simulink model "Model5DOF"  (R2020a)
settings: Solver=FixedStepAuto  StartTime=0.0  StopTime=200  FixedStep=0.01  RelTol=1e-3
libraries: simulink x5, vrlib x3
settings Model: Creator=DaseonHong  LastModifiedBy=fdcl

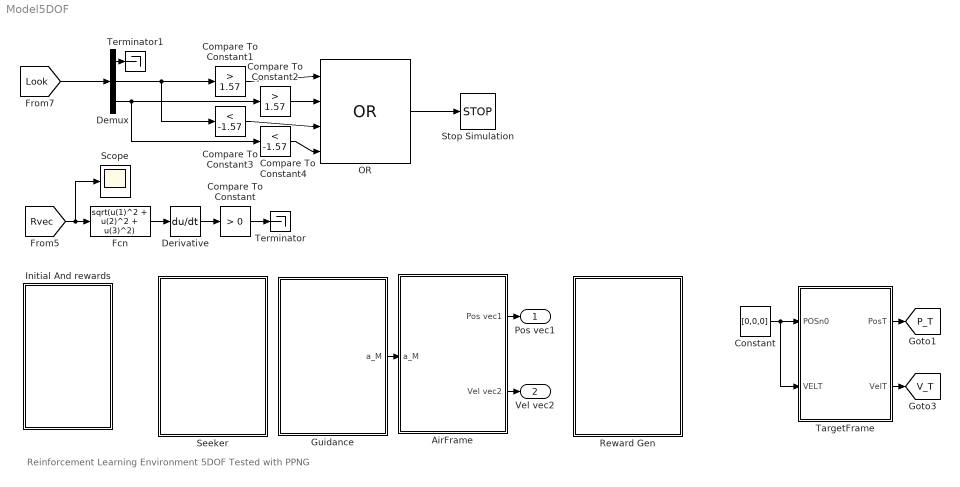
== system Model5DOF ==
  note: Reinforcement Learning Environment
      | 5DOF
      | Tested with PPNG
  AirFrame : Subsystem
  Compare To Constant : simulink/Logic and Bit Operations/Compare To Constant  relop=>  const=0  OutDataTypeStr=boolean
  Compare To Constant1 : simulink/Logic and Bit Operations/Compare To Constant  relop=>  const=1.57  OutDataTypeStr=boolean
  Compare To Constant2 : simulink/Logic and Bit Operations/Compare To Constant  relop=>  const=1.57  OutDataTypeStr=boolean
  Compare To Constant3 : simulink/Logic and Bit Operations/Compare To Constant  relop=<  const=-1.57  OutDataTypeStr=boolean
  Compare To Constant4 : simulink/Logic and Bit Operations/Compare To Constant  relop=<  const=-1.57  OutDataTypeStr=boolean
  Constant : Constant  Value=[0,0,0]
  Demux : Demux  Outputs=3
  Derivative : Derivative
  Fcn : Fcn  Expr=sqrt(u(1)^2 + u(2)^2 + u(3)^2)
  Guidance : Subsystem
  Initial And rewards : Subsystem  mask{Parameter1=90, Parameter2=10, Parameter5=10000, Parameter6=10000, Parameter7=0, Parameter8=0, Parameter4=280, Parameter15=3, Parameter9=-10000, Parameter10=5000, Parameter19=-1000, Parameter21=0, Parameter11=280, Parameter16=3, Parameter12=0, Parameter13=0, Parameter20=-1000, Parameter23=0}
      mask prompts: Parameter1 "Impact time"; Parameter2 "delayed fire"; Parameter5 "targetposx"; Parameter6 "targetposy"; Parameter7 "targetvelx"; Parameter8 "targetvely"; Parameter4 "speed"; Parameter15 "PNGcoeff"; Parameter9 "initposx"; Parameter10 "initposy"; Parameter19 "initposz"; Parameter21 "initpsi"; Parameter11 "speed"; Parameter16 "PNGcoeff"; Parameter12 "initposx"; Parameter13 "initposy"; Parameter20 "initposz"; Parameter23 "initpsi"
      mask init:
      | td      = Parameter1;
      | LaunchD = Parameter2;
      | x_t     = Parameter5;
      | y_t     = Parameter6;
      | vx_t    = Parameter7;
      | vy_t    = Parameter8;
      | 
      | SoM     = Parameter4;
      | Nval    = Parameter15;
      | x_m1    = Parameter9;
      | y_m1    = Parameter10;
      | z_m1    = Parameter19;
      | psi0    = Parameter21;
      | 
      | SoM2    = Parameter11;
      | Nval2   = Parameter16;
      | x_m2    = Parameter12;
      | y_m2    = Parameter13;
      | z_m2    = Parameter20;
      | psi20   = Parameter23;
      mask TypeOptions Parameter15: 1 | 2 | 3 | 4 | 5
      mask TypeOptions Parameter16: 1 | 2 | 3 | 4 | 5
      mask DialogControl Container4 Prompt: Common Param
      mask DialogControl Container7 Prompt: Time
      mask DialogControl Container11 Prompt: Target
      mask DialogControl Container5 Prompt: Missile 1
      mask DialogControl Container8 Prompt: Missile 2
  OR : Logic  Operator=OR  Inputs=4  IconShape=distinctive  AllPortsSameDT=off  OutDataTypeStr=boolean
  Reward Gen : Subsystem
  Scope : Scope
  Seeker : Subsystem
  Stop Simulation : Stop
  TargetFrame : Subsystem
      mask Display: image('$imagefile'); % Use "Edit Image" on toolstrip to change.
  Terminator : Terminator
  Terminator1 : Terminator
  Pos vec1 : Outport  VectorParamsAs1DForOutWhenUnconnected=off
  Vel vec2 : Outport  Port=2  VectorParamsAs1DForOutWhenUnconnected=off
  tag scope: P_T=global, V_T=global
  wires:
  Guidance/1(a_M) -> AirFrame/1(a_M)
  AirFrame/1(Pos vec1) -> Pos vec1/1
  AirFrame/2(Vel vec2) -> Vel vec2/1
  TargetFrame/2(VelT) -> [V_T]
  Constant/1 -> TargetFrame/2(VELT), TargetFrame/1(POSn0)
  TargetFrame/1(PosT) -> [P_T]
  [Rvec] -> Scope/1, Fcn/1
  Fcn/1 -> Derivative/1
  Compare To Constant/1 -> Terminator/1
  Derivative/1 -> Compare To Constant/1
  [Look] -> Demux/1
  Demux/1 -> Terminator1/1
  Demux/2 -> Compare To Constant3/1, Compare To Constant1/1
  Compare To Constant1/1 -> OR/1
  Compare To Constant2/1 -> OR/2
  Demux/3 -> Compare To Constant2/1, Compare To Constant4/1
  OR/1 -> Stop Simulation/1
  Compare To Constant3/1 -> OR/3
  Compare To Constant4/1 -> OR/4

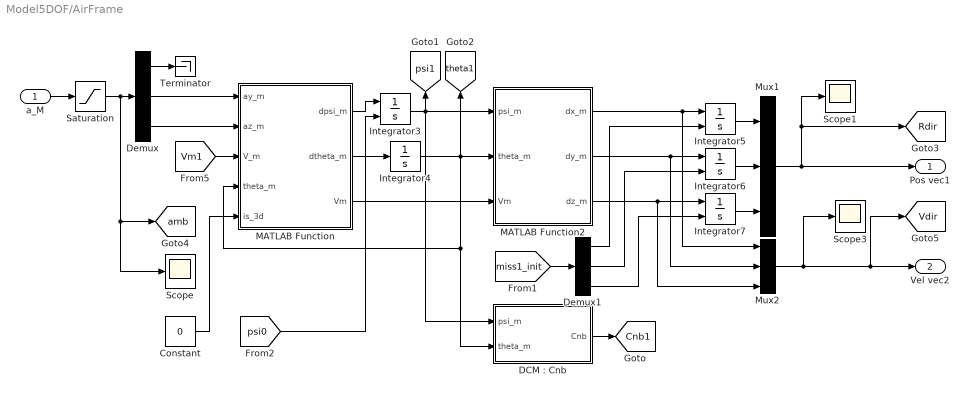
== system Model5DOF/AirFrame ==
  a_M : Inport
  Constant : Constant  Value=0
  "DCM : Cnb" : MATLAB Function  TreatAsAtomicUnit=on
  Demux : Demux  Outputs=3
  Demux1 : Demux  Outputs=3
  Integrator{3,5..7} (4 alike) : Integrator  InitialConditionSource=external
  Integrator4 : Integrator
  MATLAB Function : MATLAB Function  TreatAsAtomicUnit=on
  MATLAB Function2 : MATLAB Function  TreatAsAtomicUnit=on
  Mux1 : Mux  Inputs=3
  Mux2 : Mux  Inputs=3
  Saturation : Saturate  UpperLimit=[0;99;99]  LowerLimit=[0;-99;-99]  LinearizeAsGain=off  ZeroCross=off
  Scope : Scope
  Scope1 : Scope
  Scope3 : Scope
  Terminator : Terminator
  Pos vec1 : Outport  VectorParamsAs1DForOutWhenUnconnected=off
  Vel vec2 : Outport  Port=2  VectorParamsAs1DForOutWhenUnconnected=off
  tag scope: Cnb1=global, Rdir=global, Vdir=global, amb=global, psi1=global, theta1=global
  wires:
  MATLAB Function/1(dpsi_m) -> Integrator3/1
  Integrator7/1 -> Mux1/3
  "DCM : Cnb"/1(Cnb) -> [Cnb1]
  Constant/1 -> MATLAB Function/5(is_3d)
  [Vm1] -> MATLAB Function/3(V_m)
  Mux2/1 -> [Vdir], Vel vec2/1, Scope3/1
  Demux1/3 -> Integrator7/2
  Saturation/1 -> [amb], Scope/1, Demux/1
  Demux/3 -> MATLAB Function/2(az_m)
  MATLAB Function/3(Vm) -> MATLAB Function2/3(Vm)
  [psi0] -> Integrator3/2
  MATLAB Function/2(dtheta_m) -> Integrator4/1
  Integrator5/1 -> Mux1/1
  Demux1/2 -> Integrator6/2
  MATLAB Function2/2(dy_m) -> Mux2/2, Integrator6/1
  Demux/2 -> MATLAB Function/1(ay_m)
  Integrator3/1 -> "DCM : Cnb"/1(psi_m), MATLAB Function2/1(psi_m), [psi1]
  MATLAB Function2/3(dz_m) -> Mux2/3, Integrator7/1
  Integrator4/1 -> "DCM : Cnb"/2(theta_m), MATLAB Function/4(theta_m), MATLAB Function2/2(theta_m), [theta1]
  MATLAB Function2/1(dx_m) -> Mux2/1, Integrator5/1
  [miss1_init] -> Demux1/1
  Demux/1 -> Terminator/1
  a_M/1 -> Saturation/1
  Integrator6/1 -> Mux1/2
  Mux1/1 -> Scope1/1, [Rdir], Pos vec1/1
  Demux1/1 -> Integrator5/2

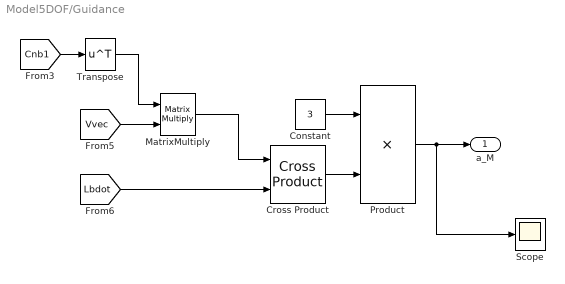
== system Model5DOF/Guidance ==
  Constant : Constant  Value=3
  Cross Product : vrlib/Utilities/Cross Product
  MatrixMultiply : Product  Multiplication=Matrix(*)
  Product : Product
  Scope : Scope
  Transpose : Math  Operator=transpose  SaturateOnIntegerOverflow=on
  a_M : Outport
  wires:
  Product/1 -> Scope/1, a_M/1
  [Vvec] -> MatrixMultiply/2
  Cross Product/1 -> Product/2
  Constant/1 -> Product/1
  [Lbdot] -> Cross Product/2
  [Cnb1] -> Transpose/1
  Transpose/1 -> MatrixMultiply/1
  MatrixMultiply/1 -> Cross Product/1

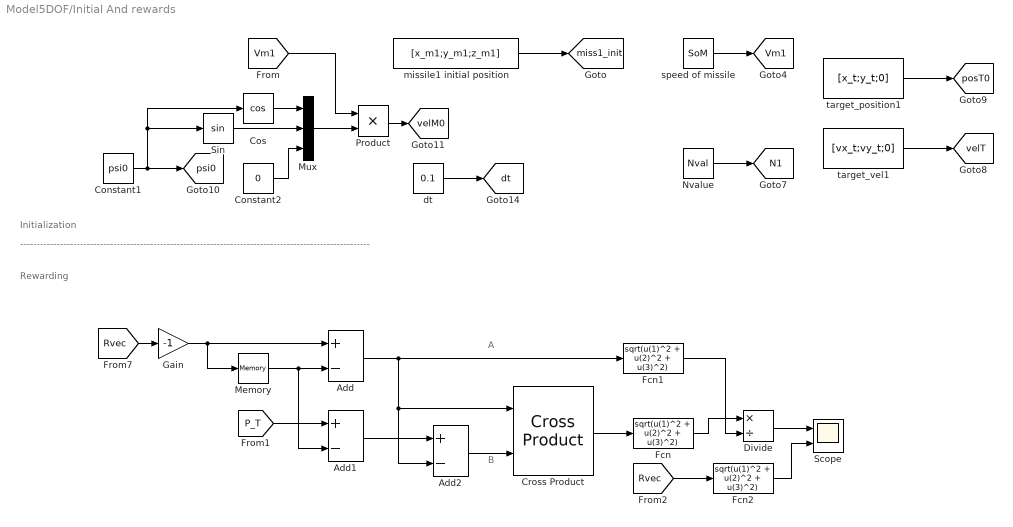
== system Model5DOF/Initial And rewards ==
  note: A
  note: Initialization
  note: ---------------------------------------------------------------------------------------------------------
  note: Rewarding
  note: B
  Add : Sum  Inputs=+-
  Add1 : Sum  Inputs=+-
  Add2 : Sum  Inputs=+-
  Constant1 : Constant  Value=psi0
  Constant2 : Constant  Value=0
  Cos : Trigonometry  Operator=cos
  Cross Product : vrlib/Utilities/Cross Product
  Divide : Product  Inputs=*/
  Fcn : Fcn  Expr=sqrt(u(1)^2 + u(2)^2 + u(3)^2)
  Fcn1 : Fcn  Expr=sqrt(u(1)^2 + u(2)^2 + u(3)^2)
  Fcn2 : Fcn  Expr=sqrt(u(1)^2 + u(2)^2 + u(3)^2)
  Gain : Gain  Gain=-1
  Memory : Memory  InitialCondition=[x_m1;y_m1;z_m1]  LinearizeAsDelay=on
  Mux : Mux  Inputs=3
  Nvalue : Constant  Value=Nval
  Product : Product
  Scope : Scope  NumInputPorts=2
  Sin : Trigonometry
  dt : Constant  Value=0.1
  missile1 initial position : Constant  Value=[x_m1;y_m1;z_m1]
  speed of missile : Constant  Value=SoM
  target_position1 : Constant  Value=[x_t;y_t;0]
  target_vel1 : Constant  Value=[vx_t;vy_t;0]
  tag scope: N1=global, Vm1=global, dt=global, miss1_init=global, posT0=global, psi0=global, velM0=global, velT=global
  wires:
  target_vel1/1 -> [velT]
  target_position1/1 -> [posT0]
  speed of missile/1 -> [Vm1]
  Nvalue/1 -> [N1]
  missile1 initial position/1 -> [miss1_init]
  Constant1/1 -> [psi0], Cos/1, Sin/1
  Mux/1 -> Product/2
  [Vm1] -> Product/1
  Sin/1 -> Mux/2
  Cos/1 -> Mux/1
  Product/1 -> [velM0]
  Constant2/1 -> Mux/3
  dt/1 -> [dt]
  [Rvec] -> Gain/1
  Gain/1 -> Add/1, Memory/1
  Memory/1 -> Add1/2, Add/2
  [P_T] -> Add1/1
  Add1/1 -> Add2/1
  Add/1 -> Cross Product/1, Add2/2, Fcn1/1
  Add2/1 -> Cross Product/2
  Cross Product/1 -> Fcn/1
  Fcn/1 -> Divide/1
  Fcn1/1 -> Divide/2
  Divide/1 -> Scope/1
  [Rvec] -> Fcn2/1
  Fcn2/1 -> Scope/2

== system Model5DOF/Reward Gen ==

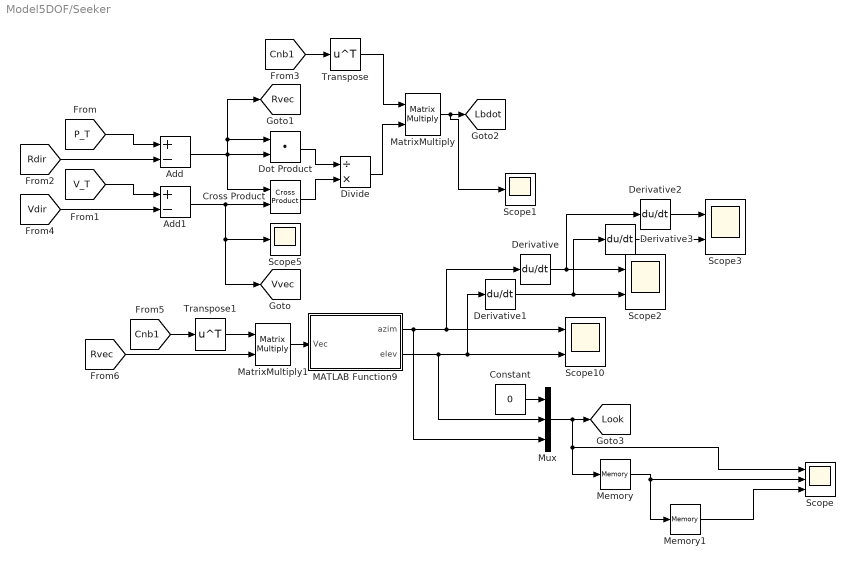
== system Model5DOF/Seeker ==
  Add : Sum  Inputs=+-
  Add1 : Sum  Inputs=+-
  Constant : Constant  Value=0
  Cross Product : vrlib/Utilities/Cross Product
  Derivative{,1..3} (4 alike) : Derivative
  Divide : Product  Inputs=/*
  Dot Product : DotProduct  InputSameDT=on  OutDataTypeStr=Inherit: Inherit via internal rule
  MATLAB Function9 : MATLAB Function  TreatAsAtomicUnit=on
  MatrixMultiply : Product  Multiplication=Matrix(*)
  MatrixMultiply1 : Product  Multiplication=Matrix(*)
  Memory : Memory  LinearizeAsDelay=on
  Memory1 : Memory  LinearizeAsDelay=on
  Mux : Mux  Inputs=3
  Scope : Scope  NumInputPorts=3
  Scope1 : Scope
  Scope10 : Scope  NumInputPorts=2
  Scope2 : Scope  NumInputPorts=2
  Scope3 : Scope  NumInputPorts=2
  Scope5 : Scope
  Transpose : Math  Operator=transpose  SaturateOnIntegerOverflow=on
  Transpose1 : Math  Operator=transpose  SaturateOnIntegerOverflow=on
  tag scope: Lbdot=global, Look=global, Rvec=global, Vvec=global
  wires:
  Dot Product/1 -> Divide/1
  Add/1 -> Cross Product/1, Dot Product/2, [Rvec], Dot Product/1
  [P_T] -> Add/1
  Add1/1 -> Cross Product/2, [Vvec], Scope5/1
  Cross Product/1 -> Divide/2
  [V_T] -> Add1/1
  [Rdir] -> Add/2
  [Vdir] -> Add1/2
  [Cnb1] -> Transpose/1
  Transpose/1 -> MatrixMultiply/1
  Divide/1 -> MatrixMultiply/2
  MatrixMultiply/1 -> Scope1/1, [Lbdot]
  MATLAB Function9/2(elev) -> Mux/2, Derivative1/1, Scope10/2
  MATLAB Function9/1(azim) -> Mux/3, Derivative/1, Scope10/1
  [Cnb1] -> Transpose1/1
  Transpose1/1 -> MatrixMultiply1/1
  MatrixMultiply1/1 -> MATLAB Function9/1(Vec)
  [Rvec] -> MatrixMultiply1/2
  Derivative/1 -> Derivative2/1, Scope2/1
  Derivative1/1 -> Derivative3/1, Scope2/2
  Derivative2/1 -> Scope3/1
  Derivative3/1 -> Scope3/2
  Constant/1 -> Mux/1
  Mux/1 -> Scope/1, Memory/1, [Look]
  Memory/1 -> Memory1/1, Scope/2
  Memory1/1 -> Scope/3

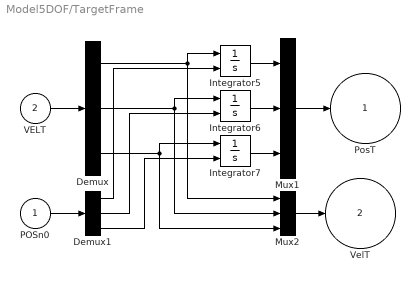
== system Model5DOF/TargetFrame ==
  POSn0 : Inport
  VELT : Inport  Port=2
  Demux : Demux  Outputs=3
  Demux1 : Demux  Outputs=3
  Integrator5 : Integrator  InitialConditionSource=external
  Integrator6 : Integrator  InitialConditionSource=external
  Integrator7 : Integrator  InitialConditionSource=external
  Mux1 : Mux  Inputs=3
  Mux2 : Mux  Inputs=3
  PosT : Outport  VectorParamsAs1DForOutWhenUnconnected=off
  VelT : Outport  Port=2  VectorParamsAs1DForOutWhenUnconnected=off
  wires:
  POSn0/1 -> Demux1/1
  Demux1/1 -> Integrator5/2
  Demux1/2 -> Integrator6/2
  Demux1/3 -> Integrator7/2
  Integrator5/1 -> Mux1/1
  Integrator6/1 -> Mux1/2
  Integrator7/1 -> Mux1/3
  Mux1/1 -> PosT/1
  Demux/2 -> Integrator6/1, Mux2/2
  Demux/3 -> Integrator7/1, Mux2/3
  Mux2/1 -> VelT/1
  Demux/1 -> Integrator5/1, Mux2/1
  VELT/1 -> Demux/1

== matlab function Model5DOF/AirFrame/DCM : Cnb ==
  data: psi_m input; Cnb output; theta_m input
function Cnb = fcn(psi_m, theta_m)

Cnb = [ cos(psi_m)*cos(theta_m),    -sin(psi_m),    cos(psi_m)*sin(theta_m);
        sin(psi_m)*cos(theta_m),    cos(psi_m),     sin(psi_m)*sin(theta_m);
        -sin(theta_m),              0,              cos(theta_m)];

end
% C_bn = [    cos(psi)*cos(the),  sin(psi)*cos(the),  -sin(the)   ;
%             -sin(psi),          cos(psi),           0           ;
%             cos(psi)*sin(the),  sin(psi)*sin(the),  cos(the)    ];

== matlab function Model5DOF/Seeker/MATLAB Function9 ==
  data: Vec input; azim output; elev output
function [azim, elev] = azim2elev(Vec)
    
    azim = atan2(Vec(2), Vec(1));
    elev = atan2(-Vec(3), sqrt(Vec(1)^2 + Vec(2)^2));

== matlab function Model5DOF/AirFrame/MATLAB Function ==
  data: ay_m input; dpsi_m output; az_m input; V_m input; theta_m input; dtheta_m output; Vm output; is_3d input
function [dpsi_m, dtheta_m, Vm] = fcn(ay_m, az_m, V_m, theta_m, is_3d)

%g = 9.81;

%dpsi_m = ay_m/(V_m*cos(theta_m));
%dtheta_m = -(az_m+g*cos(theta_m))/V_m;
%Vm = V_m;
    g = 9.81*is_3d;
    if V_m <= eps
        dpsi_m = 0;
        dtheta_m = 0;
    else
        dpsi_m = ay_m/(V_m*cos(theta_m));
        dtheta_m = -(az_m+g*cos(theta_m))/V_m;
    end
    Vm = V_m;

end

== matlab function Model5DOF/AirFrame/MATLAB Function2 ==
  settings: updateMethod=DISCRETE
  data: psi_m input; dx_m output; theta_m input; Vm input; dy_m output; dz_m output
function [dx_m, dy_m, dz_m] = fcn(psi_m, theta_m, Vm)



    dx_m = Vm*cos(psi_m)*cos(theta_m);
    dy_m = Vm*sin(psi_m)*cos(theta_m);
    dz_m = -Vm*sin(theta_m);
end
